simulink model "P1_Control_Modelo_Bloques_y_FT"  (R2021a)
settings: Solver=ode4  StartTime=0.0  StopTime=10.0  FixedStep=1e-3  RelTol=1e-3
settings Model: Creator=diego  LastModifiedBy=diego
settings SolverCC: AlgebraicLoopSolver=TrustRegion
settings DataIOCC: ReturnWorkspaceOutputs=off
settings DebuggingCC: SFMachineParentedDataDiag=warning  ArithmeticOperatorsInVariantConditions=warning
settings SFSimCC: CustomCodeUndefinedFunction=UseInterfaceOnly

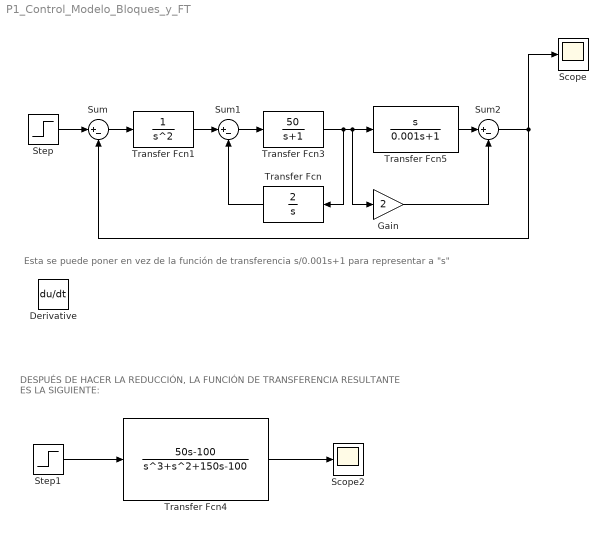
== system P1_Control_Modelo_Bloques_y_FT ==
  note: Esta se puede poner en vez de la función de transferencia s/0.001s+1 para representar a "s"
  note: DESPUÉS DE HACER LA REDUCCIÓN, LA FUNCIÓN DE TRANSFERENCIA RESULTANTE ES LA SIGUIENTE:
  Derivative : Derivative
  Gain : Gain  Gain=2
  Scope : Scope
  Scope2 : Scope
  Step : Step  SampleTime=0
  Step1 : Step  SampleTime=0
  Sum : Sum  Inputs=|+-
  Sum1 : Sum  Inputs=|+-
  Sum2 : Sum  Inputs=|+-
  Transfer Fcn : TransferFcn  Numerator=[2]  Denominator=[1 0]
  Transfer Fcn1 : TransferFcn  Denominator=[1,0,0]
  Transfer Fcn3 : TransferFcn  Numerator=[50]  Denominator=[1 1]
  Transfer Fcn4 : TransferFcn  Numerator=[50,-100]  Denominator=[1,1,150,-100]
  Transfer Fcn5 : TransferFcn  Numerator=[1 0]  Denominator=[0.001 1]
  wires:
  Step/1 -> Sum/1
  Sum/1 -> Transfer Fcn1/1
  Transfer Fcn1/1 -> Sum1/1
  Sum1/1 -> Transfer Fcn3/1
  Transfer Fcn3/1 -> Transfer Fcn/1, Gain/1, Transfer Fcn5/1
  Transfer Fcn5/1 -> Sum2/1
  Transfer Fcn/1 -> Sum1/2
  Gain/1 -> Sum2/2
  Sum2/1 -> Scope/1, Sum/2
  Step1/1 -> Transfer Fcn4/1
  Transfer Fcn4/1 -> Scope2/1
